simulink model "sim1"  (R2020b)
settings: Solver=FixedStepAuto  StartTime=0.0  StopTime=600  FixedStep=T_s  RelTol=1e-3
values from neighbouring files (symbols this model uses):
  a1 = 0.5    [lab1.m]    (also in main.m)
  A1 = 10    [lab1.m]    (also in main.m = 50)
  a2 = 1    [lab1.m]    (also in main.m = 1.5)
  A2 = 10    [lab1.m]    (also in main.m = 70)
  defuzzyfierType = defType.TS    [CAvsTS.m]    (also in ex5_A.m = defType.MoM; ex5_B.m = defType.CA; ex6_A.m = defType.CA; ex6_B_IN.m = defType.CA)
  desireValue = 30    [CAvsTS.m]    (also in ex5_A.m; ex5_B.m; ex6_A.m; ex6_B_IN.m)
  g = 9.80665    [lab1.m]    (also in main.m = 980.665)
  h1 = 50    [lab1.m]    (also in main.m = 30)
  h2 = 5    [lab1.m]    (also in main.m = 10)
  inferenceEngine = infEngine.MamdaniMinimum    [CAvsTS.m]    (also in ex5_A.m = infEngine.MamdaniProduct; ex5_B.m; ex6_A.m; ex6_B_IN.m)
  inputSetDErr = [-1 0 1]    [CAvsTS.m]    (also in ex5_A.m = [-1.5 0 1.5]; ex5_B.m; ex6_A.m = [-1.5 0 1.5]; ex6_B_IN.m = [-1.5 -0.4 0.4 1.5])
  inputSetErr = [-5 0 5]    [CAvsTS.m]    (also in ex5_A.m; ex5_B.m; ex6_A.m = [-2.5 0 2.5]; ex6_B_IN.m = [-2.5 -0.4 0.4 2.5])
  Km = 1    [lab1.m]    (also in main.m = 5)
  membershipType = memType.Triangullar    [CAvsTS.m]    (also in ex5_A.m; ex5_B.m; ex6_A.m = memType.Gaussian; ex6_B_IN.m = memType.Gaussian)
  outputSet = [-1 -0.2 0 0.2 1]    [CAvsTS.m]    (also in ex5_A.m; ex5_B.m; ex6_A.m = [-1.5 -0.2 0 0.2 1.5]; ex6_B_IN.m = [-1.5 -0.2 0 0.2 1.5])
  rho = b1/(b1+b2)    (= 0.5)    [lab1.m]
  satValue = 220    [lab1.m]    (also in main.m)
settings Model: Creator=lindt  LastModifiedBy=lindt
settings DebuggingCC: UnderSpecifiedDimensionMsg=warning

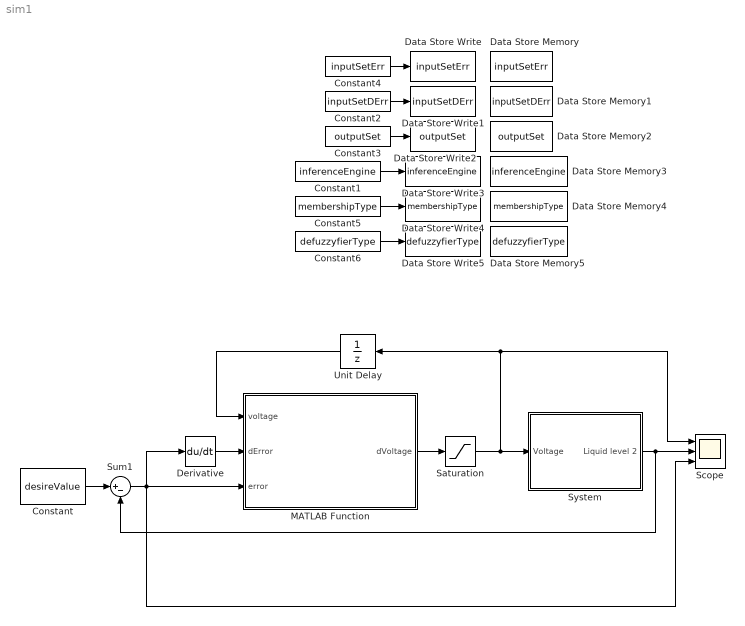
== system sim1 ==
  Constant : Constant  Value=desireValue
  Constant1 : Constant  Value=inferenceEngine
  Constant2 : Constant  Value=inputSetDErr
  Constant3 : Constant  Value=outputSet
  Constant4 : Constant  Value=inputSetErr
  Constant5 : Constant  Value=membershipType
  Constant6 : Constant  Value=defuzzyfierType
  Data Store Memory : DataStoreMemory  DataStoreName=inputSetErr  ReadBeforeWriteMsg=warning  WriteAfterWriteMsg=warning  WriteAfterReadMsg=warning  InitialValue=inputSetErr  ShowAdditionalParam=off  OutDataTypeStr=double
  Data Store Memory1 : DataStoreMemory  DataStoreName=inputSetDErr  ReadBeforeWriteMsg=warning  WriteAfterWriteMsg=warning  WriteAfterReadMsg=warning  InitialValue=inputSetDErr  ShowAdditionalParam=off  OutDataTypeStr=double
  Data Store Memory2 : DataStoreMemory  DataStoreName=outputSet  InitialValue=outputSet  ShowAdditionalParam=off  OutDataTypeStr=double
  Data Store Memory3 : DataStoreMemory  DataStoreName=inferenceEngine  ReadBeforeWriteMsg=warning  WriteAfterWriteMsg=warning  WriteAfterReadMsg=warning  InitialValue=inferenceEngine  ShowAdditionalParam=off  OutDataTypeStr=double
  Data Store Memory4 : DataStoreMemory  DataStoreName=membershipType  ReadBeforeWriteMsg=warning  WriteAfterWriteMsg=warning  WriteAfterReadMsg=warning  InitialValue=membershipType  ShowAdditionalParam=off  OutDataTypeStr=double
  Data Store Memory5 : DataStoreMemory  DataStoreName=defuzzyfierType  ReadBeforeWriteMsg=warning  WriteAfterWriteMsg=warning  WriteAfterReadMsg=warning  InitialValue=defuzzyfierType  ShowAdditionalParam=off  OutDataTypeStr=double
  Data Store Write : DataStoreWrite  DataStoreName=inputSetErr
  Data Store Write1 : DataStoreWrite  DataStoreName=inputSetDErr
  Data Store Write2 : DataStoreWrite  DataStoreName=outputSet
  Data Store Write3 : DataStoreWrite  DataStoreName=inferenceEngine
  Data Store Write4 : DataStoreWrite  DataStoreName=membershipType
  Data Store Write5 : DataStoreWrite  DataStoreName=defuzzyfierType
  Derivative : Derivative
  MATLAB Function : MATLAB Function  TreatAsAtomicUnit=on
  Saturation : Saturate  UpperLimit=satValue  LowerLimit=0
  Scope : Scope  NumInputPorts=3
  Sum1 : Sum  Inputs=|+-
  System : Subsystem
  Unit Delay : UnitDelay  SampleTime=-1  HasFrameUpgradeWarning=on
  wires:
  System/1(Liquid level 2) -> Scope/2, Sum1/2
  MATLAB Function/1(dVoltage) -> Saturation/1
  Unit Delay/1 -> MATLAB Function/1(voltage)
  Saturation/1 -> Scope/1, Unit Delay/1, System/1(Voltage)
  Derivative/1 -> MATLAB Function/2(dError)
  Constant/1 -> Sum1/1
  Sum1/1 -> Derivative/1, Scope/3, MATLAB Function/3(error)
  Constant6/1 -> Data Store Write5/1
  Constant4/1 -> Data Store Write/1
  Constant5/1 -> Data Store Write4/1
  Constant1/1 -> Data Store Write3/1
  Constant3/1 -> Data Store Write2/1
  Constant2/1 -> Data Store Write1/1

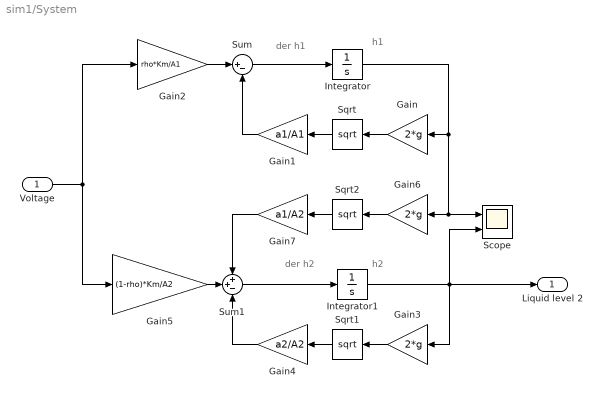
== system sim1/System ==
  note: der h1
  note: h1
  note: der h2
  note: h2
  Voltage : Inport
  Gain : Gain  Gain=2*g
  Gain1 : Gain  Gain=a1/A1
  Gain2 : Gain  Gain=rho*Km/A1
  Gain3 : Gain  Gain=2*g
  Gain4 : Gain  Gain=a2/A2
  Gain5 : Gain  Gain=(1-rho)*Km/A2
  Gain6 : Gain  Gain=2*g
  Gain7 : Gain  Gain=a1/A2
  Integrator : Integrator  InitialCondition=h1
  Integrator1 : Integrator  InitialCondition=h2
  Scope : Scope  NumInputPorts=2
  Sqrt : Sqrt  SaturateOnIntegerOverflow=on
  Sqrt1 : Sqrt  SaturateOnIntegerOverflow=on
  Sqrt2 : Sqrt  SaturateOnIntegerOverflow=on
  Sum : Sum  Inputs=|+-
  Sum1 : Sum  Inputs=++-
  Liquid level 2 : Outport
  wires:
  Gain4/1 -> Sum1/3
  Integrator1/1 -> Gain3/1, Liquid level 2/1, Scope/2
  Sqrt/1 -> Gain1/1
  Sqrt1/1 -> Gain4/1
  Gain6/1 -> Sqrt2/1
  Gain2/1 -> Sum/1
  Gain1/1 -> Sum/2
  Integrator/1 -> Gain/1, Gain6/1, Scope/1
  Gain7/1 -> Sum1/1
  Sqrt2/1 -> Gain7/1
  Sum/1 -> Integrator/1
  Voltage/1 -> Gain5/1, Gain2/1
  Gain3/1 -> Sqrt1/1
  Gain/1 -> Sqrt/1
  Gain5/1 -> Sum1/2
  Sum1/1 -> Integrator1/1

== matlab function sim1/MATLAB Function ==
  settings: updateMethod=DISCRETE  sampleTime=T_s
  data: voltage input size=1; dError input size=1; error input size=1; dVoltage output size=1; inputSetErr data_store_memory; inputSetDErr data_store_memory; outputSet data_store_memory; inferenceEngine data_store_memory; membershipType data_store_memory; defuzzyfierType data_store_memory
function dVoltage  = FuzzyController(voltage, dError, error)
%%  work 1: deadline: 16.11.2020
%%  work 2: deadline: 15.12.2020

global inputSetErr inputSetDErr outputSet
global inferenceEngine membershipType defuzzyfierType

infEngine = 'Mamdani minimum';
memType = 'Triangullar';
defType = 'CA';

switch inferenceEngine
    case 1
        infEngine = 'Mamdani minimum';
    case 2
        infEngine = 'Mamdani product';
end
switch membershipType
    case 1
        memType = 'Triangullar';
    case 2
        memType = 'Gaussian';
end
switch defuzzyfierType
    case 1
        defType = 'SoM';
    case 2
        defType = 'MoM';
    case 3
        defType = 'LoM';
    case 4
        defType = 'CA';
    case 5
        defType = 'CoG';
end


%%  if then rules - Mamdani minimum, Mamdani product
DOM = IfThenRules(error, dError, inputSetErr, inputSetDErr, infEngine, memType, max(size(outputSet)));

%%  defuzzyfier - SoM, MoM, LoM, CoG, CA
changeVoltage = defuzzyfier(DOM, outputSet, defType, memType);

%%  output - change of voltage
dVoltage = voltage(1) + changeVoltage(1);
